simulink model "model_5_exact"  (R2021b)
settings: Solver=VariableStepAuto  StartTime=0.0  StopTime=4e8
values from neighbouring files (symbols this model uses):
  att_Gains = [1 1 1]    [initial_sim2.m]
  Force_Vectors = [Force_Vectors;normal_vector]    [ellip_force_test.m]    (also in initial_sim.m = Force_Vectors'; initial_sim2.m = Force_Vectors'; multi_sim.m = Force_Vectors'; multi_sim2.m = Force_Vectors')
  max_f = 100000    [initial_sim.m]    (also in initial_sim2.m = 10)
  max_M_available = max_M_available*0.7    [initial_sim.m]    (also in initial_sim2.m; multi_sim.m; multi_sim2.m)
  mee_0 = oe2mee([a_0 e_0 incl_0 omega_0 RA_0 theta_0],p.mu)'    [Sample_OT.m]    (also in initial_sim.m = oe2mee(oe_0,params.mu)'; initial_sim2.m = oe2mp(oe_0))
  mee_f = oe2mee([a_f e_f incl_f omega_f RA_f theta_f],p.mu)'    [Sample_OT.m]    (also in initial_sim.m = oe2mee(oe_f,params.mu)'; initial_sim2.m = oe2mp(oe_f))
  Moment_Vectors = [Moment_Vectors;cross([x y z],normal_vector)]    [ellip_force_test.m]    (also in initial_sim.m = Moment_Vectors'; initial_sim2.m = Moment_Vectors'; multi_sim.m = Moment_Vectors'; multi_sim2.m = Moment_Vectors')
  N_sat = length(azimuths)    [ellip_force_test.m]    (also in initial_sim.m = 30; initial_sim2.m = 25; multi_sim.m = sim_data.N_sat; multi_sim2.m = sim_data.N_sat)
  params = 0    [Combo_OT.m]
  R_stop = 1e-2    (= 0.01)    [initial_sim2.m]
  rot_Gains = [1 1 1]    [initial_sim2.m]    (also in multi_sim2.m = inputArg(i_par,4*N_sat+6:4*N_sat+8))
  W = [6.4966    2.6843    0.7051    1.8764    3.9369]    [initial_sim2.m]    (also in lambert_pro.m = 4/(4 - Td); multi_sim2.m = inputArg(i_par,4*N_sat+1:4*N_sat+5))
undefined symbols (not defined in the file or in its folder): t_wait
libraries: slpidlib x6, simulink x3, shared6dof x2
settings Model: Creator=Mehdi  LastModifiedBy=Mehdi
settings DebuggingCC: AlgebraicLoopMsg=none

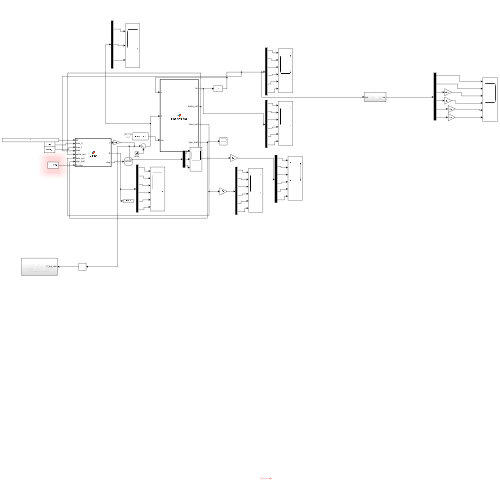
[thumbnail: Simulink's stored preview of the top-level diagram]
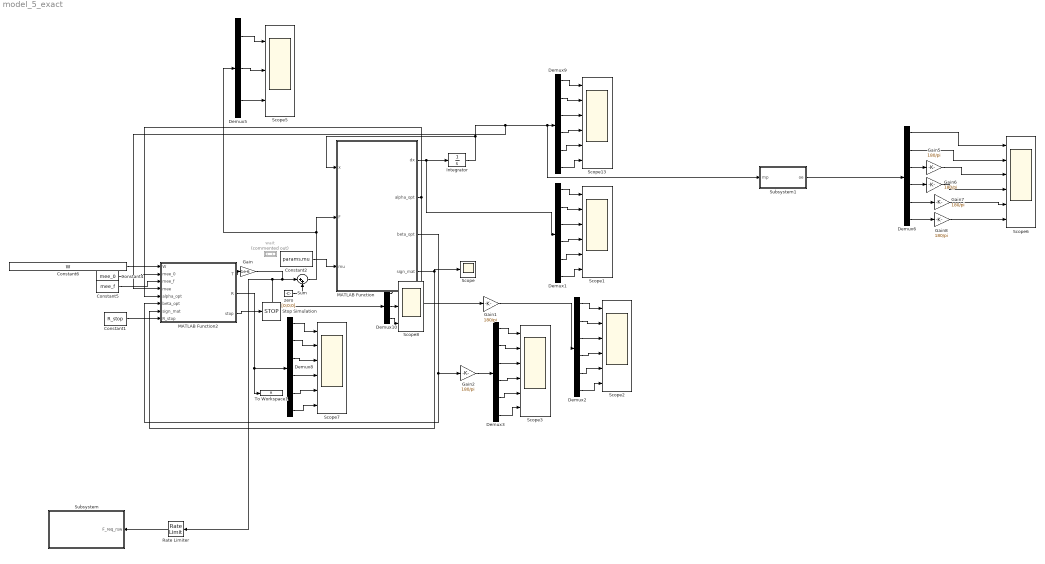
== system model_5_exact ==
  Constant1 : Constant  Value=R_stop
  Constant2 : Constant  Value=params.mu
  Constant4 : Constant  Value=mee_0
  Constant5 : Constant  Value=mee_f
  Constant6 : Constant  Value=W
  Demux{1..3,6,8..9} (6 alike) : Demux  Outputs=6
  Demux10 : Demux  Outputs=3
  Demux5 : Demux  Outputs=3
  Gain : Gain  Gain=1e-6
  Gain{1..2,5..8} (6 alike) : Gain  Gain=180/pi
  Integrator : Integrator  InitialCondition=mee_0
  MATLAB Function : MATLAB Function  TreatAsAtomicUnit=on
  MATLAB Function2 : MATLAB Function  TreatAsAtomicUnit=on
  Rate Limiter : RateLimiter  RisingSlewLimit=1e-5  FallingSlewLimit=-1e-5  SampleTimeMode=inherited
  Scope : Scope
  Scope{1..3,6..7,13} (6 alike) : Scope  NumInputPorts=6
  Scope5 : Scope  NumInputPorts=3
  Scope8 : Scope  NumInputPorts=3
  Stop Simulation : Stop
  Subsystem : Subsystem
  Subsystem1 : Subsystem
  Sum : Sum  Inputs=|++
  To Workspace1 : ToWorkspace  VariableName=R  SaveFormat=Timeseries  SampleTime=-1
      settings: MaxDataPoints=1
  wait : Subsystem  Commented=on
  zero : Constant  Value=[0;0;0]
  wires:
  Integrator/1 -> MATLAB Function2/4(mee), Subsystem1/1(mp), Demux9/1, MATLAB Function/1(x)
  Constant2/1 -> MATLAB Function/3(mu)
  Demux9/5 -> Scope13/5
  Demux9/1 -> Scope13/1
  Demux9/4 -> Scope13/4
  Demux9/3 -> Scope13/3
  Demux9/2 -> Scope13/2
  Demux9/6 -> Scope13/6
  Demux1/6 -> Scope1/6
  Demux1/2 -> Scope1/2
  Demux1/3 -> Scope1/3
  Demux1/4 -> Scope1/4
  Demux1/1 -> Scope1/1
  Demux1/5 -> Scope1/5
  Demux2/6 -> Scope2/6
  Demux2/2 -> Scope2/2
  Demux2/3 -> Scope2/3
  Demux2/4 -> Scope2/4
  Demux2/1 -> Scope2/1
  Demux2/5 -> Scope2/5
  MATLAB Function/2(alpha_opt) -> MATLAB Function2/5(alpha_opt), Gain1/1
  MATLAB Function/3(beta_opt) -> MATLAB Function2/6(beta_opt), Gain2/1
  Demux3/5 -> Scope3/5
  Demux3/1 -> Scope3/1
  Demux3/4 -> Scope3/4
  Demux3/3 -> Scope3/3
  Demux3/2 -> Scope3/2
  Demux3/6 -> Scope3/6
  Constant4/1 -> MATLAB Function2/2(mee_0)
  Constant5/1 -> MATLAB Function2/3(mee_f)
  Constant6/1 -> MATLAB Function2/1(W)
  Demux5/3 -> Scope5/3
  Demux5/2 -> Scope5/2
  Demux5/1 -> Scope5/1
  MATLAB Function2/1(T) -> Gain/1
  zero/1 -> Sum/2
  MATLAB Function2/3(stop) -> Stop Simulation/1
  Demux6/6 -> Gain8/1
  Demux6/3 -> Gain5/1
  Demux6/4 -> Gain6/1
  Demux6/5 -> Gain7/1
  Demux8/4 -> Scope7/4
  Demux8/3 -> Scope7/3
  Demux8/5 -> Scope7/5
  Demux8/2 -> Scope7/2
  Demux8/6 -> Scope7/6
  Demux8/1 -> Scope7/1
  MATLAB Function2/2(R) -> To Workspace1/1, Demux8/1
  Gain1/1 -> Demux2/1
  MATLAB Function/1(dx) -> Demux1/1, Integrator/1
  Gain2/1 -> Demux3/1
  Demux6/1 -> Scope6/1
  Demux6/2 -> Scope6/2
  Gain5/1 -> Scope6/3
  Gain6/1 -> Scope6/4
  Gain7/1 -> Scope6/5
  Gain8/1 -> Scope6/6
  Demux10/2 -> Scope8/2
  Demux10/1 -> Scope8/1
  Demux10/3 -> Scope8/3
  ? -> ?
  Sum/1 -> MATLAB Function/2(F), Demux5/1
  MATLAB Function/4(sign_mat) -> Scope/1, MATLAB Function2/7(sign_mat)
  Rate Limiter/1 -> Subsystem/1(F_req_rsw)
  Subsystem1/1(oe) -> Demux6/1
  Gain/1 -> Rate Limiter/1, Demux10/1, Sum/1
  Constant1/1 -> MATLAB Function2/8(R_stop)

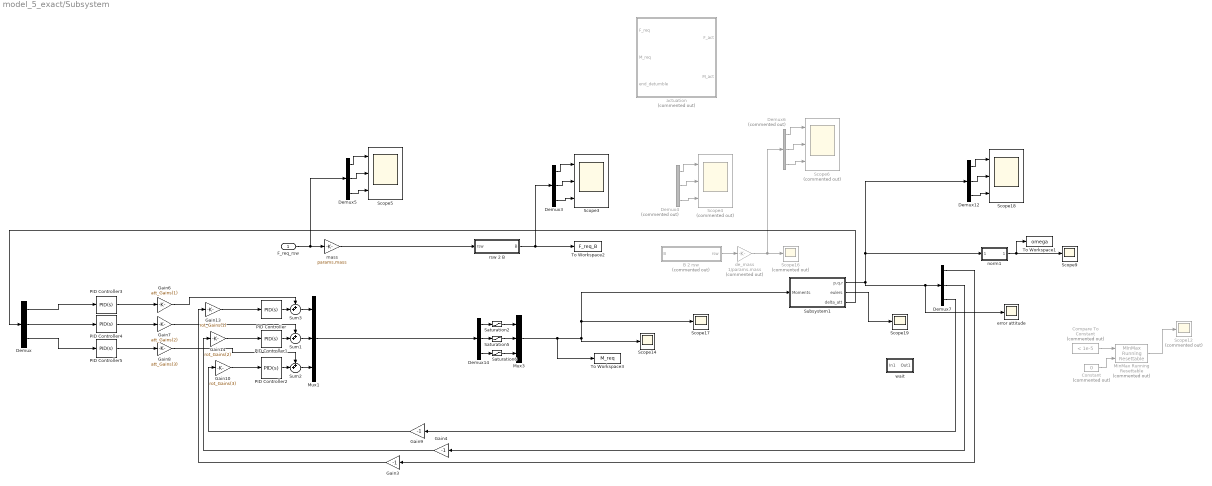
== system model_5_exact/Subsystem ==
  F_req_rsw : Inport
  B 2 rsw : Subsystem  Commented=on
  Compare To Constant : simulink/Logic and Bit Operations/Compare To Constant  Commented=on  relop=<  const=1e-5  OutDataTypeStr=boolean
  Constant : Constant  Commented=on  Value=0
  Demux{,3,5,7,12,14} (6 alike) : Demux  Outputs=3
  Demux4 : Demux  Commented=on  Outputs=3
  Demux6 : Demux  Commented=on  Outputs=3
  Gain10 : Gain  Gain=rot_Gains(3)
  Gain13 : Gain  Gain=rot_Gains(1)
  Gain14 : Gain  Gain=rot_Gains(2)
  Gain3 : Gain  Gain=-1
  Gain4 : Gain  Gain=-1
  Gain6 : Gain  Gain=att_Gains(1)
  Gain7 : Gain  Gain=att_Gains(2)
  Gain8 : Gain  Gain=att_Gains(3)
  Gain9 : Gain  Gain=-1
  MinMax Running Resettable : simulink/Math Operations/MinMax Running Resettable  Commented=on  Function=max  vinit=0.0
  Mux1 : Mux  Inputs=3
  Mux3 : Mux  Inputs=3
  PID Controller : slpidlib/PID Controller  Controller=PID  Form=Parallel  TimeDomain=Continuous-time  UseExternalTs=off  SampleTime=-1  IntegratorMethod=Forward Euler  FilterMethod=Forward Euler  ControllerParametersSource=internal  P=46047.8602202051  I=0.386669360831826  D=-40642086.1977214  UseFilter=on  N=0.0011330092652278  TunerSelectOption=Transfer Function Based (PID Tuner App)  InitialConditionSource=internal  InitialConditionForIntegrator=0  InitialConditionForFilter=0  DifferentiatorICPrevScaledInput=0  ExternalReset=none  TrackingMode=off  Kt=1  LimitOutput=off  SatLimitsSource=internal  UpperSaturationLimit=inf  LowerSaturationLimit=-inf  LinearizeAsGain=on  AntiWindupMode=none  Kb=1  POutMin=[]  POutMax=[]  IOutMin=[]  IOutMax=[]  DOutMin=[]  DOutMax=[]  NOutMin=[]  NOutMax=[]  SumOutMin=[]  SumOutMax=[]  SaturationOutMin=[]  SaturationOutMax=[]  PParamMin=[]  PParamMax=[]  IParamMin=[]  IParamMax=[]  DParamMin=[]  DParamMax=[]  NParamMin=[]  NParamMax=[]  KbParamMin=[]  KbParamMax=[]  KtParamMin=[]  KtParamMax=[]  KbOutMin=[]  KbOutMax=[]  KtOutMin=[]  KtOutMax=[]  IntegratorOutMin=[]  IntegratorOutMax=[]  FilterOutMin=[]  FilterOutMax=[]  SumI1OutMin=[]  SumI1OutMax=[]  SumI2OutMin=[]  SumI2OutMax=[]  SumI3OutMin=[]  SumI3OutMax=[]  SumI4OutMin=[]  SumI4OutMax=[]  SumDOutMin=[]  SumDOutMax=[]  DifferentiatorOutMin=[]  DifferentiatorOutMax=[]  FilterDiffOutCoefMin=[]  FilterDiffOutCoefMax=[]  ReciprocalOutMin=[]  ReciprocalOutMax=[]  SumDenOutMin=[]  SumDenOutMax=[]  SumNumOutMin=[]  SumNumOutMax=[]  DivideOutMin=[]  DivideOutMax=[]  UdiffTsProdOutMin=[]  UdiffTsProdOutMax=[]  NTsProdOutMin=[]  NTsProdOutMax=[]  UintegralTsProdOutMin=[]  UintegralTsProdOutMax=[]  UngainTsProdOutMin=[]  UngainTsProdOutMax=[]  IntegratorContinuousStateAttributes=''  IntegratorStateMustResolveToSignalObject=off  IntegratorRTWStateStorageClass=Auto  FilterContinuousStateAttributes=''  FilterStateMustResolveToSignalObject=off  FilterRTWStateStorageClass=Auto  ParallelPVariant=InternalParameters  IdealPVariant=Disabled  IVariant=InternalParameters  DVariant=InternalParameters  IntegratorVariant=Continuous  SatVariant=Disabled  AWVariant=Passthrough  PCopyVariant=Disabled  TRVariant=Disabled  FdbkBlocksVariant=Forward  IdealPFdbkVariant=Disabled  SatFdbkVariant=Disabled  DerivativeFilterVariant=ContFilter  NVariant=InternalParameters  NCopyVariant=Disabled  FilterICVariant=InternalICsFilter  IntegratorICVariant=InternalICs  ExternalResetVariant=Disabled  TRSumVariant=Passthrough  SumFdbkVariant=Disabled  SumVariant=Sum_PID  TsampFilterVariant=InternalTs  TsampNgainVariant=Passthrough  TsampIntegralVariant=Passthrough  ExternalSaturationOutDataTypeStr=Inherit: Same as second input
  PID Controller1 : slpidlib/PID Controller  Controller=PID  Form=Parallel  TimeDomain=Continuous-time  UseExternalTs=off  SampleTime=-1  IntegratorMethod=Forward Euler  FilterMethod=Forward Euler  ControllerParametersSource=internal  P=22665.0700482182  I=0.192665771971189  D=-23536701.4498255  UseFilter=on  N=0.00096296713864237  TunerSelectOption=Transfer Function Based (PID Tuner App)  InitialConditionSource=internal  InitialConditionForIntegrator=0  InitialConditionForFilter=0  DifferentiatorICPrevScaledInput=0  ExternalReset=none  TrackingMode=off  Kt=1  LimitOutput=off  SatLimitsSource=internal  UpperSaturationLimit=inf  LowerSaturationLimit=-inf  LinearizeAsGain=on  AntiWindupMode=none  Kb=1  POutMin=[]  POutMax=[]  IOutMin=[]  IOutMax=[]  DOutMin=[]  DOutMax=[]  NOutMin=[]  NOutMax=[]  SumOutMin=[]  SumOutMax=[]  SaturationOutMin=[]  SaturationOutMax=[]  PParamMin=[]  PParamMax=[]  IParamMin=[]  IParamMax=[]  DParamMin=[]  DParamMax=[]  NParamMin=[]  NParamMax=[]  KbParamMin=[]  KbParamMax=[]  KtParamMin=[]  KtParamMax=[]  KbOutMin=[]  KbOutMax=[]  KtOutMin=[]  KtOutMax=[]  IntegratorOutMin=[]  IntegratorOutMax=[]  FilterOutMin=[]  FilterOutMax=[]  SumI1OutMin=[]  SumI1OutMax=[]  SumI2OutMin=[]  SumI2OutMax=[]  SumI3OutMin=[]  SumI3OutMax=[]  SumI4OutMin=[]  SumI4OutMax=[]  SumDOutMin=[]  SumDOutMax=[]  DifferentiatorOutMin=[]  DifferentiatorOutMax=[]  FilterDiffOutCoefMin=[]  FilterDiffOutCoefMax=[]  ReciprocalOutMin=[]  ReciprocalOutMax=[]  SumDenOutMin=[]  SumDenOutMax=[]  SumNumOutMin=[]  SumNumOutMax=[]  DivideOutMin=[]  DivideOutMax=[]  UdiffTsProdOutMin=[]  UdiffTsProdOutMax=[]  NTsProdOutMin=[]  NTsProdOutMax=[]  UintegralTsProdOutMin=[]  UintegralTsProdOutMax=[]  UngainTsProdOutMin=[]  UngainTsProdOutMax=[]  IntegratorContinuousStateAttributes=''  IntegratorStateMustResolveToSignalObject=off  IntegratorRTWStateStorageClass=Auto  FilterContinuousStateAttributes=''  FilterStateMustResolveToSignalObject=off  FilterRTWStateStorageClass=Auto  ParallelPVariant=InternalParameters  IdealPVariant=Disabled  IVariant=InternalParameters  DVariant=InternalParameters  IntegratorVariant=Continuous  SatVariant=Disabled  AWVariant=Passthrough  PCopyVariant=Disabled  TRVariant=Disabled  FdbkBlocksVariant=Forward  IdealPFdbkVariant=Disabled  SatFdbkVariant=Disabled  DerivativeFilterVariant=ContFilter  NVariant=InternalParameters  NCopyVariant=Disabled  FilterICVariant=InternalICsFilter  IntegratorICVariant=InternalICs  ExternalResetVariant=Disabled  TRSumVariant=Passthrough  SumFdbkVariant=Disabled  SumVariant=Sum_PID  TsampFilterVariant=InternalTs  TsampNgainVariant=Passthrough  TsampIntegralVariant=Passthrough  ExternalSaturationOutDataTypeStr=Inherit: Same as second input
  PID Controller2 : slpidlib/PID Controller  Controller=PID  Form=Parallel  TimeDomain=Continuous-time  UseExternalTs=off  SampleTime=-1  IntegratorMethod=Forward Euler  FilterMethod=Forward Euler  ControllerParametersSource=internal  P=57156.0298545842  I=0.0195126142821294  D=-17592936910.7499  UseFilter=on  N=3.24050294010588e-06  TunerSelectOption=Transfer Function Based (PID Tuner App)  InitialConditionSource=internal  InitialConditionForIntegrator=0  InitialConditionForFilter=0  DifferentiatorICPrevScaledInput=0  ExternalReset=none  TrackingMode=off  Kt=1  LimitOutput=off  SatLimitsSource=internal  UpperSaturationLimit=inf  LowerSaturationLimit=-inf  LinearizeAsGain=on  AntiWindupMode=none  Kb=1  POutMin=[]  POutMax=[]  IOutMin=[]  IOutMax=[]  DOutMin=[]  DOutMax=[]  NOutMin=[]  NOutMax=[]  SumOutMin=[]  SumOutMax=[]  SaturationOutMin=[]  SaturationOutMax=[]  PParamMin=[]  PParamMax=[]  IParamMin=[]  IParamMax=[]  DParamMin=[]  DParamMax=[]  NParamMin=[]  NParamMax=[]  KbParamMin=[]  KbParamMax=[]  KtParamMin=[]  KtParamMax=[]  KbOutMin=[]  KbOutMax=[]  KtOutMin=[]  KtOutMax=[]  IntegratorOutMin=[]  IntegratorOutMax=[]  FilterOutMin=[]  FilterOutMax=[]  SumI1OutMin=[]  SumI1OutMax=[]  SumI2OutMin=[]  SumI2OutMax=[]  SumI3OutMin=[]  SumI3OutMax=[]  SumI4OutMin=[]  SumI4OutMax=[]  SumDOutMin=[]  SumDOutMax=[]  DifferentiatorOutMin=[]  DifferentiatorOutMax=[]  FilterDiffOutCoefMin=[]  FilterDiffOutCoefMax=[]  ReciprocalOutMin=[]  ReciprocalOutMax=[]  SumDenOutMin=[]  SumDenOutMax=[]  SumNumOutMin=[]  SumNumOutMax=[]  DivideOutMin=[]  DivideOutMax=[]  UdiffTsProdOutMin=[]  UdiffTsProdOutMax=[]  NTsProdOutMin=[]  NTsProdOutMax=[]  UintegralTsProdOutMin=[]  UintegralTsProdOutMax=[]  UngainTsProdOutMin=[]  UngainTsProdOutMax=[]  IntegratorContinuousStateAttributes=''  IntegratorStateMustResolveToSignalObject=off  IntegratorRTWStateStorageClass=Auto  FilterContinuousStateAttributes=''  FilterStateMustResolveToSignalObject=off  FilterRTWStateStorageClass=Auto  ParallelPVariant=InternalParameters  IdealPVariant=Disabled  IVariant=InternalParameters  DVariant=InternalParameters  IntegratorVariant=Continuous  SatVariant=Disabled  AWVariant=Passthrough  PCopyVariant=Disabled  TRVariant=Disabled  FdbkBlocksVariant=Forward  IdealPFdbkVariant=Disabled  SatFdbkVariant=Disabled  DerivativeFilterVariant=ContFilter  NVariant=InternalParameters  NCopyVariant=Disabled  FilterICVariant=InternalICsFilter  IntegratorICVariant=InternalICs  ExternalResetVariant=Disabled  TRSumVariant=Passthrough  SumFdbkVariant=Disabled  SumVariant=Sum_PID  TsampFilterVariant=InternalTs  TsampNgainVariant=Passthrough  TsampIntegralVariant=Passthrough  ExternalSaturationOutDataTypeStr=Inherit: Same as second input
  PID Controller3 : slpidlib/PID Controller  Controller=PID  Form=Parallel  TimeDomain=Continuous-time  UseExternalTs=off  SampleTime=-1  IntegratorMethod=Forward Euler  FilterMethod=Forward Euler  ControllerParametersSource=internal  P=7.2870758510925  I=4.81330185008632e-05  D=272296.627551547  UseFilter=on  N=0.00293249740535471  TunerSelectOption=Transfer Function Based (PID Tuner App)  InitialConditionSource=internal  InitialConditionForIntegrator=0  InitialConditionForFilter=0  DifferentiatorICPrevScaledInput=0  ExternalReset=none  TrackingMode=off  Kt=1  LimitOutput=off  SatLimitsSource=internal  UpperSaturationLimit=inf  LowerSaturationLimit=-inf  LinearizeAsGain=on  AntiWindupMode=none  Kb=1  POutMin=[]  POutMax=[]  IOutMin=[]  IOutMax=[]  DOutMin=[]  DOutMax=[]  NOutMin=[]  NOutMax=[]  SumOutMin=[]  SumOutMax=[]  SaturationOutMin=[]  SaturationOutMax=[]  PParamMin=[]  PParamMax=[]  IParamMin=[]  IParamMax=[]  DParamMin=[]  DParamMax=[]  NParamMin=[]  NParamMax=[]  KbParamMin=[]  KbParamMax=[]  KtParamMin=[]  KtParamMax=[]  KbOutMin=[]  KbOutMax=[]  KtOutMin=[]  KtOutMax=[]  IntegratorOutMin=[]  IntegratorOutMax=[]  FilterOutMin=[]  FilterOutMax=[]  SumI1OutMin=[]  SumI1OutMax=[]  SumI2OutMin=[]  SumI2OutMax=[]  SumI3OutMin=[]  SumI3OutMax=[]  SumI4OutMin=[]  SumI4OutMax=[]  SumDOutMin=[]  SumDOutMax=[]  DifferentiatorOutMin=[]  DifferentiatorOutMax=[]  FilterDiffOutCoefMin=[]  FilterDiffOutCoefMax=[]  ReciprocalOutMin=[]  ReciprocalOutMax=[]  SumDenOutMin=[]  SumDenOutMax=[]  SumNumOutMin=[]  SumNumOutMax=[]  DivideOutMin=[]  DivideOutMax=[]  UdiffTsProdOutMin=[]  UdiffTsProdOutMax=[]  NTsProdOutMin=[]  NTsProdOutMax=[]  UintegralTsProdOutMin=[]  UintegralTsProdOutMax=[]  UngainTsProdOutMin=[]  UngainTsProdOutMax=[]  IntegratorContinuousStateAttributes=''  IntegratorStateMustResolveToSignalObject=off  IntegratorRTWStateStorageClass=Auto  FilterContinuousStateAttributes=''  FilterStateMustResolveToSignalObject=off  FilterRTWStateStorageClass=Auto  ParallelPVariant=InternalParameters  IdealPVariant=Disabled  IVariant=InternalParameters  DVariant=InternalParameters  IntegratorVariant=Continuous  SatVariant=Disabled  AWVariant=Passthrough  PCopyVariant=Disabled  TRVariant=Disabled  FdbkBlocksVariant=Forward  IdealPFdbkVariant=Disabled  SatFdbkVariant=Disabled  DerivativeFilterVariant=ContFilter  NVariant=InternalParameters  NCopyVariant=Disabled  FilterICVariant=InternalICsFilter  IntegratorICVariant=InternalICs  ExternalResetVariant=Disabled  TRSumVariant=Passthrough  SumFdbkVariant=Disabled  SumVariant=Sum_PID  TsampFilterVariant=InternalTs  TsampNgainVariant=Passthrough  TsampIntegralVariant=Passthrough  ExternalSaturationOutDataTypeStr=Inherit: Same as second input
  PID Controller4 : slpidlib/PID Controller  Controller=PID  Form=Parallel  TimeDomain=Continuous-time  UseExternalTs=off  SampleTime=-1  IntegratorMethod=Forward Euler  FilterMethod=Forward Euler  ControllerParametersSource=internal  P=7.2870758510925  I=4.81330185008632e-05  D=272296.627551547  UseFilter=on  N=0.00293249740535471  TunerSelectOption=Transfer Function Based (PID Tuner App)  InitialConditionSource=internal  InitialConditionForIntegrator=0  InitialConditionForFilter=0  DifferentiatorICPrevScaledInput=0  ExternalReset=none  TrackingMode=off  Kt=1  LimitOutput=off  SatLimitsSource=internal  UpperSaturationLimit=inf  LowerSaturationLimit=-inf  LinearizeAsGain=on  AntiWindupMode=none  Kb=1  POutMin=[]  POutMax=[]  IOutMin=[]  IOutMax=[]  DOutMin=[]  DOutMax=[]  NOutMin=[]  NOutMax=[]  SumOutMin=[]  SumOutMax=[]  SaturationOutMin=[]  SaturationOutMax=[]  PParamMin=[]  PParamMax=[]  IParamMin=[]  IParamMax=[]  DParamMin=[]  DParamMax=[]  NParamMin=[]  NParamMax=[]  KbParamMin=[]  KbParamMax=[]  KtParamMin=[]  KtParamMax=[]  KbOutMin=[]  KbOutMax=[]  KtOutMin=[]  KtOutMax=[]  IntegratorOutMin=[]  IntegratorOutMax=[]  FilterOutMin=[]  FilterOutMax=[]  SumI1OutMin=[]  SumI1OutMax=[]  SumI2OutMin=[]  SumI2OutMax=[]  SumI3OutMin=[]  SumI3OutMax=[]  SumI4OutMin=[]  SumI4OutMax=[]  SumDOutMin=[]  SumDOutMax=[]  DifferentiatorOutMin=[]  DifferentiatorOutMax=[]  FilterDiffOutCoefMin=[]  FilterDiffOutCoefMax=[]  ReciprocalOutMin=[]  ReciprocalOutMax=[]  SumDenOutMin=[]  SumDenOutMax=[]  SumNumOutMin=[]  SumNumOutMax=[]  DivideOutMin=[]  DivideOutMax=[]  UdiffTsProdOutMin=[]  UdiffTsProdOutMax=[]  NTsProdOutMin=[]  NTsProdOutMax=[]  UintegralTsProdOutMin=[]  UintegralTsProdOutMax=[]  UngainTsProdOutMin=[]  UngainTsProdOutMax=[]  IntegratorContinuousStateAttributes=''  IntegratorStateMustResolveToSignalObject=off  IntegratorRTWStateStorageClass=Auto  FilterContinuousStateAttributes=''  FilterStateMustResolveToSignalObject=off  FilterRTWStateStorageClass=Auto  ParallelPVariant=InternalParameters  IdealPVariant=Disabled  IVariant=InternalParameters  DVariant=InternalParameters  IntegratorVariant=Continuous  SatVariant=Disabled  AWVariant=Passthrough  PCopyVariant=Disabled  TRVariant=Disabled  FdbkBlocksVariant=Forward  IdealPFdbkVariant=Disabled  SatFdbkVariant=Disabled  DerivativeFilterVariant=ContFilter  NVariant=InternalParameters  NCopyVariant=Disabled  FilterICVariant=InternalICsFilter  IntegratorICVariant=InternalICs  ExternalResetVariant=Disabled  TRSumVariant=Passthrough  SumFdbkVariant=Disabled  SumVariant=Sum_PID  TsampFilterVariant=InternalTs  TsampNgainVariant=Passthrough  TsampIntegralVariant=Passthrough  ExternalSaturationOutDataTypeStr=Inherit: Same as second input
  PID Controller5 : slpidlib/PID Controller  Controller=PID  Form=Parallel  TimeDomain=Continuous-time  UseExternalTs=off  SampleTime=-1  IntegratorMethod=Forward Euler  FilterMethod=Forward Euler  ControllerParametersSource=internal  P=7.2870758510925  I=4.81330185008632e-05  D=272296.627551547  UseFilter=on  N=0.00293249740535471  TunerSelectOption=Transfer Function Based (PID Tuner App)  InitialConditionSource=internal  InitialConditionForIntegrator=0  InitialConditionForFilter=0  DifferentiatorICPrevScaledInput=0  ExternalReset=none  TrackingMode=off  Kt=1  LimitOutput=off  SatLimitsSource=internal  UpperSaturationLimit=inf  LowerSaturationLimit=-inf  LinearizeAsGain=on  AntiWindupMode=none  Kb=1  POutMin=[]  POutMax=[]  IOutMin=[]  IOutMax=[]  DOutMin=[]  DOutMax=[]  NOutMin=[]  NOutMax=[]  SumOutMin=[]  SumOutMax=[]  SaturationOutMin=[]  SaturationOutMax=[]  PParamMin=[]  PParamMax=[]  IParamMin=[]  IParamMax=[]  DParamMin=[]  DParamMax=[]  NParamMin=[]  NParamMax=[]  KbParamMin=[]  KbParamMax=[]  KtParamMin=[]  KtParamMax=[]  KbOutMin=[]  KbOutMax=[]  KtOutMin=[]  KtOutMax=[]  IntegratorOutMin=[]  IntegratorOutMax=[]  FilterOutMin=[]  FilterOutMax=[]  SumI1OutMin=[]  SumI1OutMax=[]  SumI2OutMin=[]  SumI2OutMax=[]  SumI3OutMin=[]  SumI3OutMax=[]  SumI4OutMin=[]  SumI4OutMax=[]  SumDOutMin=[]  SumDOutMax=[]  DifferentiatorOutMin=[]  DifferentiatorOutMax=[]  FilterDiffOutCoefMin=[]  FilterDiffOutCoefMax=[]  ReciprocalOutMin=[]  ReciprocalOutMax=[]  SumDenOutMin=[]  SumDenOutMax=[]  SumNumOutMin=[]  SumNumOutMax=[]  DivideOutMin=[]  DivideOutMax=[]  UdiffTsProdOutMin=[]  UdiffTsProdOutMax=[]  NTsProdOutMin=[]  NTsProdOutMax=[]  UintegralTsProdOutMin=[]  UintegralTsProdOutMax=[]  UngainTsProdOutMin=[]  UngainTsProdOutMax=[]  IntegratorContinuousStateAttributes=''  IntegratorStateMustResolveToSignalObject=off  IntegratorRTWStateStorageClass=Auto  FilterContinuousStateAttributes=''  FilterStateMustResolveToSignalObject=off  FilterRTWStateStorageClass=Auto  ParallelPVariant=InternalParameters  IdealPVariant=Disabled  IVariant=InternalParameters  DVariant=InternalParameters  IntegratorVariant=Continuous  SatVariant=Disabled  AWVariant=Passthrough  PCopyVariant=Disabled  TRVariant=Disabled  FdbkBlocksVariant=Forward  IdealPFdbkVariant=Disabled  SatFdbkVariant=Disabled  DerivativeFilterVariant=ContFilter  NVariant=InternalParameters  NCopyVariant=Disabled  FilterICVariant=InternalICsFilter  IntegratorICVariant=InternalICs  ExternalResetVariant=Disabled  TRSumVariant=Passthrough  SumFdbkVariant=Disabled  SumVariant=Sum_PID  TsampFilterVariant=InternalTs  TsampNgainVariant=Passthrough  TsampIntegralVariant=Passthrough  ExternalSaturationOutDataTypeStr=Inherit: Same as second input
  Saturation2 : Saturate  UpperLimit=max_M_available(1,1)  LowerLimit=max_M_available(1,2)
  Saturation5 : Saturate  UpperLimit=max_M_available(2,1)  LowerLimit=max_M_available(2,2)
  Saturation6 : Saturate  UpperLimit=max_M_available(3,1)  LowerLimit=max_M_available(3,2)
  Scope12 : Scope  Commented=on
  Scope{9,14,17,19} (4 alike) : Scope
  Scope16 : Scope  Commented=on
  Scope18 : Scope  NumInputPorts=3
  Scope3 : Scope  NumInputPorts=3
  Scope4 : Scope  Commented=on  NumInputPorts=3
  Scope5 : Scope  NumInputPorts=3
  Scope6 : Scope  Commented=on  NumInputPorts=3
  Subsystem1 : Subsystem
  Sum1 : Sum  Inputs=++|
  Sum2 : Sum  Inputs=++|
  Sum3 : Sum  Inputs=++|
  To Workspace1 : ToWorkspace  VariableName=omega  SaveFormat=Timeseries  SampleTime=-1
      settings: MaxDataPoints=1
  To Workspace2 : ToWorkspace  VariableName=F_req_B  SaveFormat=Timeseries  SampleTime=-1
  To Workspace3 : ToWorkspace  VariableName=M_req  SaveFormat=Timeseries  SampleTime=-1
  actuation : Subsystem  Commented=on
  de_mass : Gain  Commented=on  Gain=1/params.mass
  error attitude : Scope
  mass : Gain  Gain=params.mass
  norm1 : Subsystem
  rsw 2 B : Subsystem
  wait : Subsystem
  wires:
  norm1/1(Out1) -> To Workspace1/1, Scope9/1
  Gain9/1 -> Gain10/1
  Gain3/1 -> Gain13/1
  Mux3/1 -> Subsystem1/1(Moments), Scope17/1, Scope14/1, To Workspace3/1
  B 2 rsw/1(rsw) -> de_mass/1
  Demux7/2 -> Gain4/1
  Saturation5/1 -> Mux3/2
  Gain4/1 -> Gain14/1
  Demux7/3 -> Gain9/1
  Demux14/3 -> Saturation6/1
  Demux12/2 -> Scope18/2
  Saturation2/1 -> Mux3/1
  Demux12/1 -> Scope18/1
  rsw 2 B/1(B) -> To Workspace2/1, Demux3/1
  Subsystem1/2(eulers) -> Scope19/1
  Demux14/1 -> Saturation2/1
  Demux12/3 -> Scope18/3
  Demux14/2 -> Saturation5/1
  MinMax Running Resettable/1 -> Scope12/1
  Compare To Constant/1 -> MinMax Running Resettable/1
  Constant/1 -> MinMax Running Resettable/2
  Demux7/1 -> Gain3/1
  Saturation6/1 -> Mux3/3
  Demux3/3 -> Scope3/3
  Demux3/1 -> Scope3/1
  Demux3/2 -> Scope3/2
  Demux4/2 -> Scope4/2
  Demux4/1 -> Scope4/1
  Demux4/3 -> Scope4/3
  F_req_rsw/1 -> Demux5/1, mass/1
  Demux5/2 -> Scope5/2
  Demux5/1 -> Scope5/1
  Demux5/3 -> Scope5/3
  Demux6/3 -> Scope6/3
  Demux6/1 -> Scope6/1
  Demux6/2 -> Scope6/2
  de_mass/1 -> Demux6/1, Scope16/1
  mass/1 -> rsw 2 B/1(rsw)
  Mux1/1 -> Demux14/1
  Subsystem1/1(p,q,r) -> error attitude/1, Demux7/1, Demux12/1, norm1/1(p,q,r)
  Subsystem1/3(delta_att) -> Demux/1
  Demux/1 -> PID Controller3/1
  Demux/2 -> PID Controller4/1
  Demux/3 -> PID Controller5/1
  PID Controller3/1 -> Gain6/1
  Gain6/1 -> Sum3/1
  PID Controller4/1 -> Gain7/1
  PID Controller5/1 -> Gain8/1
  PID Controller/1 -> Sum3/2
  Sum3/1 -> Mux1/1
  Gain13/1 -> PID Controller/1
  Gain14/1 -> PID Controller1/1
  Gain10/1 -> PID Controller2/1
  Gain7/1 -> Sum1/1
  Gain8/1 -> Sum2/1
  PID Controller2/1 -> Sum2/2
  Sum2/1 -> Mux1/3
  PID Controller1/1 -> Sum1/2
  Sum1/1 -> Mux1/2

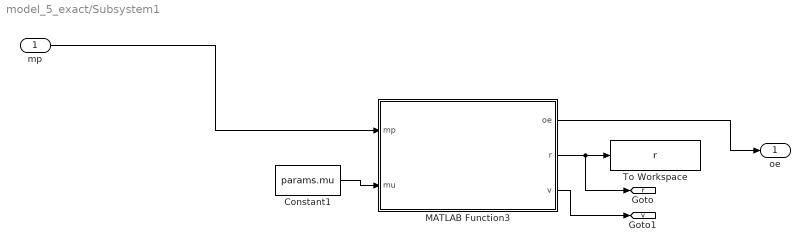
== system model_5_exact/Subsystem1 ==
  mp : Inport
  Constant1 : Constant  Value=params.mu
  MATLAB Function3 : MATLAB Function  TreatAsAtomicUnit=on
  To Workspace : ToWorkspace  VariableName=r  SaveFormat=Timeseries  SampleTime=-1
  oe : Outport
  tag scope: r=global, v=global
  wires:
  Constant1/1 -> MATLAB Function3/2(mu)
  MATLAB Function3/1(oe) -> oe/1
  MATLAB Function3/2(r) -> [r], To Workspace/1
  mp/1 -> MATLAB Function3/1(mp)
  MATLAB Function3/3(v) -> [v]

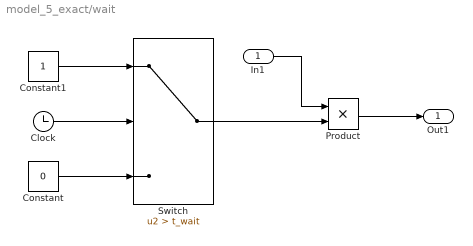
== system model_5_exact/wait ==
  In1 : Inport
  Clock : Clock
  Constant : Constant  Value=0
  Constant1 : Constant
  Product : Product
  Switch : Switch  Criteria=u2 > Threshold  Threshold=t_wait
  Out1 : Outport
  wires:
  Clock/1 -> Switch/2
  Constant1/1 -> Switch/1
  Switch/1 -> Product/2
  Product/1 -> Out1/1
  In1/1 -> Product/1
  Constant/1 -> Switch/3

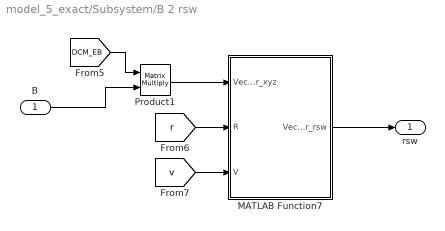
== system model_5_exact/Subsystem/B 2 rsw ==
  B : Inport
  MATLAB Function7 : MATLAB Function  TreatAsAtomicUnit=on
  Product1 : Product  Multiplication=Matrix(*)
  rsw : Outport
  wires:
  Product1/1 -> MATLAB Function7/1(Vector_xyz)
  [v] -> MATLAB Function7/3(V)
  [DCM_EB] -> Product1/1
  [r] -> MATLAB Function7/2(R)
  B/1 -> Product1/2
  MATLAB Function7/1(Vector_rsw) -> rsw/1

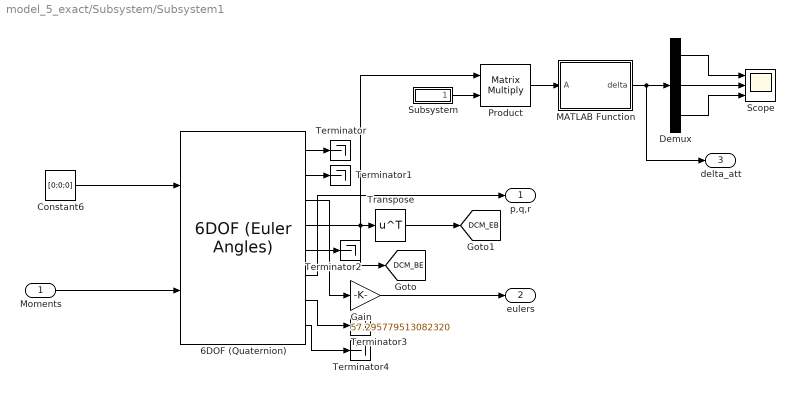
== system model_5_exact/Subsystem/Subsystem1 ==
  Moments : Inport
  6DOF (Quaternion) : shared6dof/6DOF (Euler Angles)  units=Metric (MKS)  mtype=Fixed  rep=Quaternion  xme_0=[0 0 0]  Vm_0=[0 0 0]  eul_0=eul_0  pm_0=pqr_0  mass_0=1.0  mass_e=0.5  mass_f=2.0  inertia=params.Inertia  inertia_e=eye(3)  inertia_f=2*eye(3)  k_quat=1.0  vre_flag=on  abi_flag=off  aMode=0  xme_statename=''  Vm_statename=''  eul_statename=''  quat_statename=''  pm_statename=''  mass_statename=''
      settings: SourceProductBaseCode=AE,PW,DR,MT,UV,VE
  Constant6 : Constant  Value=[0;0;0]
  Demux : Demux  Outputs=3
  Gain : Gain  Gain=57.295779513082320
  MATLAB Function : MATLAB Function  TreatAsAtomicUnit=on
  Product : Product  Multiplication=Matrix(*)
  Scope : Scope  NumInputPorts=3
  Subsystem : Subsystem
  Terminator{,1..4} (5 alike) : Terminator
  Transpose : Math  Operator=transpose  SaturateOnIntegerOverflow=on
  p,q,r : Outport
  eulers : Outport  Port=2
  delta_att : Outport  Port=3
  tag scope: DCM_BE=global, DCM_EB=global
  wires:
  6DOF (Quaternion)/7 -> Terminator3/1
  Constant6/1 -> 6DOF (Quaternion)/1
  6DOF (Quaternion)/3 -> Gain/1
  6DOF (Quaternion)/1 -> Terminator/1
  6DOF (Quaternion)/6 -> p,q,r/1
  6DOF (Quaternion)/5 -> Terminator2/1
  6DOF (Quaternion)/2 -> Terminator1/1
  Gain/1 -> eulers/1
  6DOF (Quaternion)/4 -> Product/1, [DCM_BE], Transpose/1
  6DOF (Quaternion)/8 -> Terminator4/1
  Moments/1 -> 6DOF (Quaternion)/2
  Transpose/1 -> [DCM_EB]
  Product/1 -> MATLAB Function/1(A)
  MATLAB Function/1(delta) -> delta_att/1, Demux/1
  Demux/1 -> Scope/1
  Demux/2 -> Scope/2
  Demux/3 -> Scope/3
  Subsystem/1(DCM_T') -> Product/2

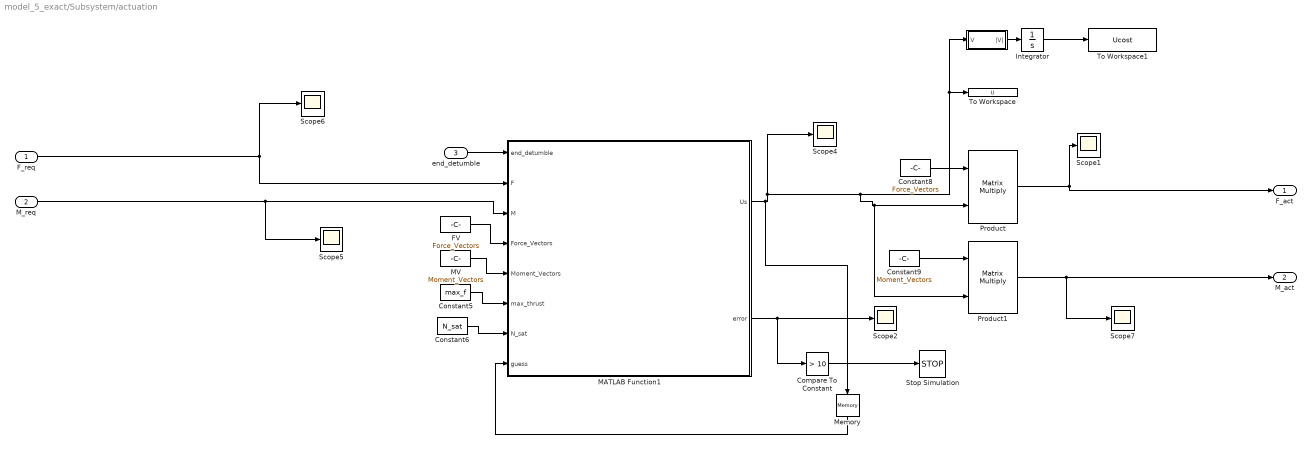
== system model_5_exact/Subsystem/actuation ==
  F_req : Inport
  M_req : Inport  Port=2
  end_detumble : Inport  Port=3
  " " : Subsystem
  Compare To Constant : simulink/Logic and Bit Operations/Compare To Constant  relop=>  const=10  OutDataTypeStr=boolean
  Constant5 : Constant  Value=max_f
  Constant6 : Constant  Value=N_sat
  Constant8 : Constant  Value=Force_Vectors
  Constant9 : Constant  Value=Moment_Vectors
  FV : Constant  Value=Force_Vectors
  Integrator : Integrator
  MATLAB Function1 : MATLAB Function  TreatAsAtomicUnit=on
  MV : Constant  Value=Moment_Vectors
  Memory : Memory  InitialCondition=zeros(N_sat,1)
  Product : Product  Multiplication=Matrix(*)
  Product1 : Product  Multiplication=Matrix(*)
  Scope{1..2,4..7} (6 alike) : Scope
  Stop Simulation : Stop
  To Workspace : ToWorkspace  VariableName=U  SaveFormat=Timeseries  SampleTime=-1
  To Workspace1 : ToWorkspace  VariableName=Ucost  SaveFormat=Timeseries  SampleTime=-1
      settings: MaxDataPoints=1
  F_act : Outport
  M_act : Outport  Port=2
  wires:
  Constant6/1 -> MATLAB Function1/7(N_sat)
  Constant9/1 -> Product1/1
  Memory/1 -> MATLAB Function1/8(guess)
  MATLAB Function1/2(error) -> Compare To Constant/1, Scope2/1
  FV/1 -> MATLAB Function1/4(Force_Vectors)
  MV/1 -> MATLAB Function1/5(Moment_Vectors)
  Product1/1 -> Scope7/1, M_act/1
  Constant8/1 -> Product/1
  Constant5/1 -> MATLAB Function1/6(max_thrust)
  F_req/1 -> MATLAB Function1/2(F), Scope6/1
  Product/1 -> F_act/1, Scope1/1
  end_detumble/1 -> MATLAB Function1/1(end_detumble)
  MATLAB Function1/1(Us) -> Scope4/1, Product/2, Product1/2, " "/1(V), To Workspace/1, Memory/1
  " "/1(|V|) -> Integrator/1
  Integrator/1 -> To Workspace1/1
  M_req/1 -> MATLAB Function1/3(M), Scope5/1
  Compare To Constant/1 -> Stop Simulation/1

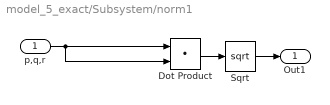
== system model_5_exact/Subsystem/norm1 ==
  p,q,r : Inport
  Dot Product : DotProduct  InputSameDT=on  OutDataTypeStr=Inherit: Inherit via internal rule
  Sqrt : Sqrt  OutputSignalType=real  SaturateOnIntegerOverflow=on
  Out1 : Outport
  wires:
  Dot Product/1 -> Sqrt/1
  p,q,r/1 -> Dot Product/1, Dot Product/2
  Sqrt/1 -> Out1/1

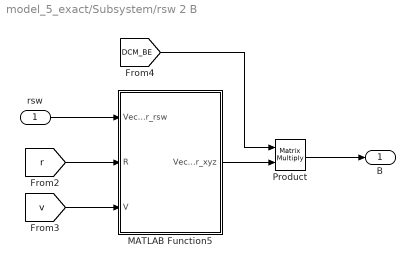
== system model_5_exact/Subsystem/rsw 2 B ==
  rsw : Inport
  MATLAB Function5 : MATLAB Function  TreatAsAtomicUnit=on
  Product : Product  Multiplication=Matrix(*)
  B : Outport
  wires:
  [DCM_BE] -> Product/1
  rsw/1 -> MATLAB Function5/1(Vector_rsw)
  MATLAB Function5/1(Vector_xyz) -> Product/2
  [v] -> MATLAB Function5/3(V)
  [r] -> MATLAB Function5/2(R)
  Product/1 -> B/1

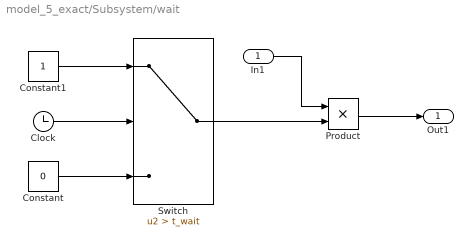
== system model_5_exact/Subsystem/wait ==
  In1 : Inport
  Clock : Clock
  Constant : Constant  Value=0
  Constant1 : Constant
  Product : Product
  Switch : Switch  Criteria=u2 > Threshold  Threshold=t_wait
  Out1 : Outport
  wires:
  Clock/1 -> Switch/2
  Constant1/1 -> Switch/1
  Switch/1 -> Product/2
  Product/1 -> Out1/1
  In1/1 -> Product/1
  Constant/1 -> Switch/3

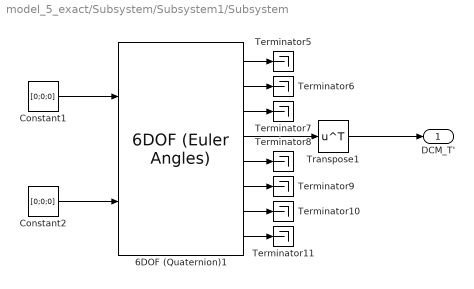
== system model_5_exact/Subsystem/Subsystem1/Subsystem ==
  6DOF (Quaternion)1 : shared6dof/6DOF (Euler Angles)  units=Metric (MKS)  mtype=Fixed  rep=Quaternion  xme_0=[0 0 0]  Vm_0=[0 0 0]  eul_0=target_angles  pm_0=[0 0 0]  mass_0=1.0  mass_e=0.5  mass_f=2.0  inertia=params.Inertia  inertia_e=eye(3)  inertia_f=2*eye(3)  k_quat=1.0  vre_flag=on  abi_flag=off  aMode=0  xme_statename=''  Vm_statename=''  eul_statename=''  quat_statename=''  pm_statename=''  mass_statename=''
      settings: SourceProductBaseCode=AE,PW,DR,MT,UV,VE
  Constant1 : Constant  Value=[0;0;0]
  Constant2 : Constant  Value=[0;0;0]
  Terminator{5..11} (7 alike) : Terminator
  Transpose1 : Math  Operator=transpose  SaturateOnIntegerOverflow=on
  DCM_T' : Outport
  wires:
  6DOF (Quaternion)1/8 -> Terminator11/1
  6DOF (Quaternion)1/3 -> Terminator7/1
  Constant1/1 -> 6DOF (Quaternion)1/1
  6DOF (Quaternion)1/6 -> Terminator9/1
  6DOF (Quaternion)1/1 -> Terminator5/1
  6DOF (Quaternion)1/7 -> Terminator10/1
  Constant2/1 -> 6DOF (Quaternion)1/2
  6DOF (Quaternion)1/5 -> Terminator8/1
  6DOF (Quaternion)1/2 -> Terminator6/1
  6DOF (Quaternion)1/4 -> Transpose1/1
  Transpose1/1 -> DCM_T'/1

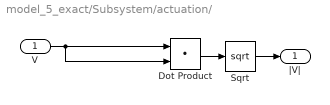
== system model_5_exact/Subsystem/actuation/  ==
  V : Inport
  Dot Product : DotProduct  InputSameDT=on  OutDataTypeStr=Inherit: Inherit via internal rule
  Sqrt : Sqrt  OutputSignalType=real  SaturateOnIntegerOverflow=on
  |V| : Outport
  wires:
  Dot Product/1 -> Sqrt/1
  V/1 -> Dot Product/1, Dot Product/2
  Sqrt/1 -> |V|/1

== matlab function model_5_exact/Subsystem/B 2 rsw/MATLAB Function7 ==
  data: Vector_xyz input; R input; Vector_rsw output; V input
function Vector_rsw=xyz2rsw(Vector_xyz,R,V)

Vector_rsw=zeros(3,1);

e_r=R/norm(R);
h=cross(R,V);
e_w=h/norm(h);
e_s=cross(e_w,e_r);


Vector_rsw(1)=dot(Vector_xyz,e_r);
Vector_rsw(2)=dot(Vector_xyz,e_s);
Vector_rsw(3)=dot(Vector_xyz,e_w);

end

== matlab function model_5_exact/Subsystem/actuation/MATLAB Function1 ==
  data: end_detumble input; F input size=3; Us output; M input size=3; Force_Vectors input; Moment_Vectors input; error output; max_thrust input; N_sat input size=1; guess input
function [Us,error] = cotrol_allocation(end_detumble,F,M,Force_Vectors,Moment_Vectors,max_thrust,N_sat,guess)


maxIter=5;

% Us=zeros(N_sat,1);
% Uss=zeros(N_sat,1);
if end_detumble==0
    %     b=[F(1);F(2);F(3);0;0;0];
    b=[F(1);F(2);F(3);M(1);M(2);M(3)];
else
    b=[F(1);F(2);F(3);0;0;0];
    %     b=[0;0;0;M(1);M(2);M(3)];
end
C=[Force_Vectors;Moment_Vectors];

options = optimoptions('lsqnonlin','Algorithm','levenberg-marquardt','MaxIterations',maxIter);
LB=zeros(N_sat,1);
UB=max_thrust*ones(N_sat,1);
% x0=zeros(N_sat,1);
x0=guess;

% C*x0-b

fun=@(x)(C*x-b);



[Uss,error]=lsqnonlin(fun,x0,LB,UB,options);


if error<1e-4
    
    
    Us=Uss(1:30,1);
    
else
    
    Us=zeros(30,1);
    
end

%
% F_out=Force_Vectors*Us;
% M_out=Moment_Vectors*Us;



% Us=C*x0-b;


% for i=1:N_sat
%     Us(i)=U1(i);
% end

% error=0;


end

== matlab function model_5_exact/MATLAB Function ==
  data: x input; F input; dx output; mu input; alpha_opt output; beta_opt output; sign_mat output
function [dx,alpha_opt,beta_opt,sign_mat] = path_dynamics(x,F,mu)


%%%% to be optimized

% a
% ep1=e*sin(omega+OMEGA);
% ep2=e*cos(omega+OMEGA);
% zig1=tan(inc/2)*sin(OMEGA);
% zig2=tan(inc/2)*cos(OMEGA);
% lambda=theta+omega+OMEGA;


a=x(1);
ep1=x(2);
ep2=x(3);
zig1=x(4);
zig2=x(5);
lambda=x(6);

slam=sin(lambda);
clam=cos(lambda);
L=a*(1-ep1^2-ep2^2);
h=sqrt(mu*L);
r=L/(1+ep1*slam+ep2*clam);

%%% to be optimized!



a_dot_=2*a^2/h*[ep2*slam-ep1*clam L/r 0];
ep1_dot_=r/h*[-L/r*clam ep1+(1+L/r)*slam -ep2*(zig1*clam-zig2*slam)];
ep2_dot_=r/h*[L/r*slam ep2+(1+L/r)*clam ep1*(zig1*clam-zig2*slam)];
zig1_dot_=r/(2*h)*[0 0 (1+zig1^2+zig2^2)*slam];
zig2_dot_=r/(2*h)*[0 0 (1+zig1^2+zig2^2)*clam];
lambda_dot_=r/h*[0 0 zig2*slam-zig1*clam];


a_dot=dot(a_dot_,F);
ep1_dot=dot(ep1_dot_,F);
ep2_dot=dot(ep2_dot_,F);
zig1_dot=dot(zig1_dot_,F);
zig2_dot=dot(zig2_dot_,F);
lambda_dot=h/r^2+dot(lambda_dot_,F);

% % % a_dot=2*a^2/h*dot([ep2*slam-ep1*clam L/r 0],F);
% % % ep1_dot=r/h*dot([-L/r*clam ep1+(1+L/r)*slam -ep2*(zig1*clam-zig2*slam)],F);
% % % ep2_dot=r/h*dot([L/r*slam ep2+(1+L/r)*clam ep1*(zig1*clam-zig2*slam)],F);
% % % zig1_dot=r/(2*h)*dot([0 0 (1+zig1^2+zig2^2)*slam],F);
% % % zig2_dot=r/(2*h)*dot([0 0 (1+zig1^2+zig2^2)*clam],F);
% % % lambda_dot=h/r^2+r/h*dot([0 0 zig2*slam-zig1*clam],F);

% dx=zeros(6,1);

dx=[a_dot;ep1_dot;ep2_dot;zig1_dot;zig2_dot;lambda_dot];


% sign_mat=sign([ep2*slam-ep1*clam L/r 0;-L/r*clam ep1+(1+L/r)*slam -ep2*(zig1*clam-zig2*slam);L/r*slam ep2+(1+L/r)*clam ep1*(zig1*clam-zig2*slam);0 0 (1+zig1^2+zig2^2)*slam;0 0 (1+zig1^2+zig2^2)*clam;0 0 zig2*slam-zig1*clam]);
% sign_mat=sign([ep2*slam-ep1*clam 1 0;-clam ep1+(1+L/r)*slam -ep2*(zig1*clam-zig2*slam);slam ep2+(1+L/r)*clam ep1*(zig1*clam-zig2*slam);0 0 slam;0 0 clam;0 0 zig2*slam-zig1*clam]);



% [a e i omega OMEGA theta]

alpha_opt=zeros(6,1);
beta_opt=zeros(6,1);


%%% based on oe
% % % ep1plus=ep1*slam+ep2*clam;
% % % ep2minus=ep2*slam-ep2*clam;
% % % zig1c=zig1*clam-zig2*slam;
% % % zig2s=zig2*slam-zig1*clam;
% % % alpha_opt(1)=atan((r/L)*ep2minus);
% % % alpha_opt(2)=atan((L/r*ep2minus)/(ep1^2+ep2^2+(1+L/r)*ep1plus));
% % % beta_opt(3)=sign(zig1*slam+zig2*clam)*pi/2;
% % % beta_opt(4)=sign(zig2s)*pi/2;
% % % alpha_opt(5)=atan(-L/(L+r)*(ep1plus/ep2minus));
% % % sinaw=sin(alpha_opt(5));
% % % cosaw=cos(alpha_opt(5));
% % % beta_opt(5)=atan((-(ep1^2+ep2^2)/(zig1^2+zig2^2))*((r*(zig1^2+zig2^2)*zig2s+r/2*(1+zig1^2+zig2^2)*zig1c)/(L*ep1plus*sinaw-(L+r)*ep2minus*cosaw)));
% alpha_opt(6)=atan(-L/(L+r)*ep1plus/ep2minus);
% beta_opt(6)=


alpha_opt(1)=atan(r/L*(ep2*slam-ep1*clam));
alpha_opt(2)=atan(-L*clam/(r*ep1+(r+L)*slam));
alpha_opt(3)=atan(L*slam/(r*ep2+(r+L)*clam));


beta_opt(2)=atan(r*ep2*(zig1*clam-zig2*slam)/(L*clam*sin(alpha_opt(2))-(r*ep1+(r+L)*slam)*cos(alpha_opt(2))));
beta_opt(3)=atan(r*ep1*(zig1*clam-zig2*slam)/(L*slam*sin(alpha_opt(3))-(r*ep2+(r+L)*clam)*cos(alpha_opt(3))));

beta_opt(4)=sign(slam)*pi/2;
beta_opt(5)=sign(clam)*pi/2;

beta_opt(6)=sign(zig2*slam-zig1*clam)*pi/2;


% e=sqrt(ep1^2+ep2^2);
% inc=2*atan(sqrt(zig1^2+zig2^2));
% OMEGA=atan(zig1/zig2);
% omega=atan(ep1/ep2)-OMEGA;
% theta=lambda-atan(ep1/ep2);

% 
% F_sample=zeros(3,6);
% sign_vec=zeros(6,2);

% for i=1:6
%     F_sample(:,i)=[sin(alpha_opt(i))*cos(beta_opt(i));cos(alpha_opt(i))*cos(beta_opt(i));sin(beta_opt(i))];
% end

% for i=1:6
%     F_sample(:,i)=[sin(alpha_opt(i));cos(alpha_opt(i));0];
% end
% 
% sign_vec(1,1)=2*a^2/h*dot([ep2*slam-ep1*clam L/r 0],F_sample(:,1));
% sign_vec(2,1)=r/h*dot([-L/r*clam ep1+(1+L/r)*slam -ep2*(zig1*clam-zig2*slam)],F_sample(:,2));
% sign_vec(3,1)=r/h*dot([L/r*slam ep2+(1+L/r)*clam ep1*(zig1*clam-zig2*slam)],F_sample(:,3));
% sign_vec(4,1)=r/(2*h)*dot([0 0 (1+zig1^2+zig2^2)*slam],F_sample(:,4));
% sign_vec(5,1)=r/(2*h)*dot([0 0 (1+zig1^2+zig2^2)*clam],F_sample(:,5));
% sign_vec(6,1)=h/r^2+r/h*dot([0 0 zig2*slam-zig1*clam],F_sample(:,6));
% 
% for i=1:6
%     F_sample(:,i)=[0;cos(beta_opt(i));sin(beta_opt(i))];
% end
% 
% 
% 
% sign_vec(1,2)=2*a^2/h*dot([ep2*slam-ep1*clam L/r 0],F_sample(:,1));
% sign_vec(2,2)=r/h*dot([-L/r*clam ep1+(1+L/r)*slam -ep2*(zig1*clam-zig2*slam)],F_sample(:,2));
% sign_vec(3,2)=r/h*dot([L/r*slam ep2+(1+L/r)*clam ep1*(zig1*clam-zig2*slam)],F_sample(:,3));
% sign_vec(4,2)=r/(2*h)*dot([0 0 (1+zig1^2+zig2^2)*slam],F_sample(:,4));
% sign_vec(5,2)=r/(2*h)*dot([0 0 (1+zig1^2+zig2^2)*clam],F_sample(:,5));
% sign_vec(6,2)=h/r^2+r/h*dot([0 0 zig2*slam-zig1*clam],F_sample(:,6));
% 
% sign_vec=sign(sign_vec);





% sign_mat=zeros(6,3);
% 
% sign_mat(1,:)=[ep2*slam-ep1*clam L/r 0];
% sign_mat(2,:)=[-L/r*clam ep1+(1+L/r)*slam -ep2*(zig1*clam-zig2*slam)];
% sign_mat(3,:)=[L/r*slam ep2+(1+L/r)*clam ep1*(zig1*clam-zig2*slam)];
% sign_mat(4,:)=[0 0 (1+zig1^2+zig2^2)*slam];
% sign_mat(5,:)=[0 0 (1+zig1^2+zig2^2)*clam];
% sign_mat(6,:)=[0 0 zig2*slam-zig1*clam];
% 
% sign_mat=sign(sign_mat);


sign_mat=sign([a_dot_;ep1_dot_;ep2_dot_;zig1_dot_;zig2_dot_;lambda_dot_]);




end

== matlab function model_5_exact/MATLAB Function2 ==
  data: W input; mee_0 input; mee_f input; mee input; alpha_opt input; beta_opt input; T output; R output; stop output; sign_mat input; R_stop input
function [T,R,stop]  = Guider(W,mee_0,mee_f,mee,alpha_opt,beta_opt,sign_mat,R_stop)


stop=0;

% mark=0;

R=zeros(6,1);


%
% ss(1)=-1;
% ss(2)=-1;
% % ss(4)=-1;

T=[0;0;0];

% for i=1:5
%
%     %     if abs(mee_f(i)-mee_0(i))>1e-5 && abs(mee_f(i)-mee(i))>1e-5
%
%     if abs(mee_f(i)-mee_0(i))>1e-5
%
%         R(i)=abs((mee(i)-mee_f(i))/(mee_f(i)-mee_0(i)));
%
%         %         if  abs(R(i))>5
%         %             R(i)=5;
%         %         end
%         %         if  abs(R(i))<-5
%         %             R(i)=-5;
%         %         end
%
%     else
%         R(i)=0;
%     end
% end


for i=1:5

    %     if abs(mee_f(i)-mee_0(i))>1e-5 && abs(mee_f(i)-mee(i))>1e-5
    %      ss(i)=sign(oe_f(i)-oe(i));

    if abs(mee_f(i)-mee_0(i))>1e-5

        R(i)=abs((mee_f(i)-mee(i))/(mee_f(i)-mee_0(i)));

        %         if  abs(R(i))>5
        %             R(i)=5;
        %         end
        %         if  abs(R(i))<-5
        %             R(i)=-5;
        %         end


    else
        R(i)=0;
    end
end



if norm(R)<R_stop
    stop=1;
end

% ss(1)=-1;

% alpha_opt1=zeros(6,1);
% beta_opt1=zeros(6,1);


alpha_opt1=alpha_opt;
beta_opt1=beta_opt;



% % % ss(1)=sign(mee_f(1)-mee(1));  %% sign ok
% % % ss(2)=-sign(mee_f(2)-mee(2));  %% sign ok
% % % ss(3)=-sign(mee_f(3)-mee(3));
% % % ss(4)=sign(mee_f(4)-mee(4));
% % % ss(5)=sign(mee_f(5)-mee(5));
% % % ss(6)=sign(mee_f(6)-mee(6));

% ss=R_dot;

% ang1=rem(x(6)+2*pi,2*pi);
% if ang1>pi
%     ss(2)=-ss(2);
% alpha_opt(2)=2*pi-alpha_opt(2);
% end

% n=0;

%
% if mee_f(1)<mee(1)
%     ss(1)=-1;
% end
%
% if mee_f(2)<mee(2)
%     ss(2)=-1;
% end

% sign_mat1=ones(6,3);

% for i=1:6
%     for j=1:3
%         if (sign_mat(i,j)<0 && mee_f(i)>mee(i)) || (sign_mat(i,j)>0 && mee_f(i)<mee(i))
%             sign_mat1(i,j)=-1;
%         end
%     end
%
% end

% for i=1:6
%         if (sign_vec(i,1)<0 && mee_f(i)>mee(i)) || (sign_vec(i,1)>0 && mee_f(i)<mee(i)) || (sign_vec(i,2)<0 && mee_f(i)>mee(i)) || (sign_vec(i,2)>0 && mee_f(i)<mee(i))
%             ss(i)=-1;
%         end
% 
% end


% for i=1:6
%     if (sign_vec(i,1)<0 && oe_f(i)>oe(i)) || (sign_vec(i,1)>0 && oe_f(i)<oe(i))
%         alpha_opt1(i)= -alpha_opt(i);
%     end
% 
%     if (sign_vec(i,2)<0 && oe_f(i)>oe(i)) || (sign_vec(i,2)>0 && oe_f(i)<oe(i))
%         beta_opt1(i)= -beta_opt(i);
%     end
% end


% for i=1:6
%     if (sign_vec(i,1)<0 && R(i)>0) || (sign_vec(i,1)>0 && R(i)<0)
%         alpha_opt1(i)= -alpha_opt(i);
%     end
% 
%     if (sign_vec(i,2)<0 && R(i)>0) || (sign_vec(i,2)>0 && R(i)<0)
%         beta_opt1(i)= -beta_opt(i);
%     end
% end

% for i=1:5
%     if sign_vec(i,1)<0
%         alpha_opt1(i)= pi+alpha_opt(i);
%     end
% 
%     if sign_vec(i,2)<0
%         beta_opt1(i)= pi+beta_opt(i);
%     end
% end



% for i=1:5
%     s1=0;
%     s2=0;
%     if (sign_vec(i,1)==-1  && mee_f(i)>mee(i)) || (sign_vec(i,1)==1 && mee_f(i)<mee(i))
% %         ss(i)=-1;
%                 alpha_opt1(i)=-alpha_opt1(i);
%         s1=1;
% 
%     end
% 
%     if (sign_vec(i,2)==-1  && mee_f(i)>mee(i)) || (sign_vec(i,2)==1 && mee_f(i)<mee(i))
% %         ss(i)=-1;
%                 beta_opt1(i)=-beta_opt1(i);
%         s2=1;
%     end
% 
%     if s1~=s2
%         mark=1;
%     end
% 
%     %     if (sign_vec(i,2)==-1  && mee_f(i)>mee(i)) || (sign_vec(i,2)==1 && mee_f(i)<mee(i))
%     %         beta_opt1(i)=pi+beta_opt1(i);
%     %     end
% end


ss_rsw=ones(6,3);

for i=1:6
    for j=1:3
        if (sign_mat(i,j)<0 && mee_f(i)>mee(i)) || (sign_mat(i,j)>0 && mee_f(i)<mee(i))
            ss_rsw(i,j)=-1;
        end
    end
end

for i=1:5

    %     n=n+1;
    %     ss=1;
    %     ang1=rem(x(6)+2*pi,2*pi);
    %     if ang1<pi
    %         alpha_opt(i)=-alpha_opt(i);
    % ss=-1;
    %     end

    %         ss=sign(x(i)-mp_f(i));
    %     ss=1;
    %
    % ss=-1;

    %     if (sign_mat(i,1)==-1  && mee_f(i)>mee(i)) || (sign_mat(i,1)==1 && mee_f(i)<mee(i))
    %         alpha_opt(i)=-abs(alpha_opt(i));
    %     else
    %         alpha_opt(i)=abs(alpha_opt(i));
    %     end
    %
    %     if (sign_mat(i,3)==-1  && mee_f(i)>mee(i)) || (sign_mat(i,3)==1 && mee_f(i)<mee(i))
    %         beta_opt(i)=-abs(beta_opt(i));
    %     else
    %         beta_opt(i)=abs(beta_opt(i));
    %     end

    %     if (sign_mat(i,1)==-1  && mee_f(i)>mee(i)) || (sign_mat(i,1)==1 && mee_f(i)<mee(i))
    %                 alpha_opt1(i)=-alpha_opt(i);
    % %         ss(i)=-1;
    %     else
    %                 alpha_opt1(i)=abs(alpha_opt(i));
    %     end
    %
    %     if (sign_mat(i,3)==-1  && mee_f(i)>mee(i)) || (sign_mat(i,3)==1 && mee_f(i)<mee(i))
    %                 beta_opt1(i)=-beta_opt(i);
    %     else
    %                 beta_opt1(i)=abs(beta_opt(i));
    %     end






%     T=T+ss(i)*W(i)*R(i)*([sin(alpha_opt1(i))*cos(beta_opt1(i));cos(alpha_opt1(i))*cos(beta_opt1(i));sin(beta_opt1(i))]);

    T=T+W(i)*R(i)*([ss_rsw(i,1)*abs(sin(alpha_opt1(i))*cos(beta_opt1(i)));ss_rsw(i,2)*abs(cos(alpha_opt1(i))*cos(beta_opt1(i)));ss_rsw(i,3)*abs(sin(beta_opt1(i)))]);

    % T=T+ss(n)*W(n)*R(i)*([sin(alpha_opt(i))*cos(0);cos(alpha_opt(i))*cos(0);sin(beta_opt(i))]);
    %
end

% for i=1:6
%     n=n+1;
%     ss=1;
%     ang1=rem(x(6)+2*pi,2*pi);
%     if ang1<pi
%         alpha_opt(i)=-alpha_opt(i);
% ss=-1;
%     end

%         ss=sign(x(i)-mp_f(i));
%     ss=1;
%
% ss=-1;
%     T=T+ss(i)*W(i)*R(i)*([sin(alpha_opt(i))*cos(beta_opt(i));cos(alpha_opt(i))*cos(beta_opt(i));sin(beta_opt(i))]);
% T=T+ss(i)*W(n)*R(i)*([sin(0)*cos(beta_opt(i));cos(0)*cos(beta_opt(i));sin(beta_opt(i))]);
%
% end

% T=T./sum(W);


T=T./sum(W);


% if norm(T)>1e-10
% 
%     T=T./norm(T);
% 
% else
%     T=[0;0;0];
% end

end

== matlab function model_5_exact/Subsystem1/MATLAB Function3 ==
  data: mp input; oe output; mu input; r output; v output
function [oe,r,v]=mp2oe(mp,mu)



oe=mp2oe(mp);

[r, v] = oe2rv(oe,mu);



% % % % a=mp(1);
% % % % ep1=mp(2);
% % % % ep2=mp(3);
% % % % zig1=mp(4);
% % % % zig2=mp(5);
% % % % lambda=mp(6);
% % % % 
% % % % 
% % % % % % ep1=e*sin(omega+OMEGA);
% % % % % % ep2=e*cos(omega+OMEGA);
% % % % % % zig1=tan(inc/2)*sin(OMEGA);
% % % % % % zig2=tan(inc/2)*cos(OMEGA);
% % % % % % lambda=theta+omega+OMEGA;
% % % % % %
% % % % % % mp=[a;ep1;ep2;zig1;zig2;lambda];
% % % % 
% % % % %%% to be optimized
% % % % e=sqrt(ep1^2+ep2^2);
% % % % inc=2*atan(sqrt(zig1^2+zig2^2));
% % % % 
% % % % if inc==0
% % % %     OMEGA=0;
% % % % else
% % % %     tan1=tan(inc/2);
% % % %     OMEGA=atan3(zig1/tan1,zig2/tan1);
% % % % end
% % % % 
% % % % 
% % % % % if sign(zig2)*sign(cos(OMEGA))<0 || sign(zig1)*sign(sin(OMEGA))<0
% % % % %     inc=-inc;
% % % % % end
% % % % 
% % % % 
% % % % if OMEGA>pi
% % % %     OMEGA=OMEGA-2*pi;
% % % % end
% % % % 
% % % % % inc=inc*(sign(zig2)*sign(cos(OMEGA)));
% % % % 
% % % % if e==0
% % % %     omega=0;
% % % % else
% % % %     omega=atan3(ep1/e,ep2/e)-OMEGA;
% % % % end
% % % % 
% % % % if omega>2*pi
% % % %     omega=omega-2*pi;
% % % %     
% % % % end
% % % % 
% % % % 
% % % % theta=lambda-omega-OMEGA;
% % % % if theta<0
% % % %     theta=theta+2*pi;
% % % % end
% % % % 
% % % % if theta>2*pi
% % % %     theta=rem(theta,2*pi);
% % % % end
% % % % 
% % % % oe=[a;e;inc;omega;OMEGA;theta];


end

== matlab function model_5_exact/Subsystem/Subsystem1/MATLAB Function ==
  data: A input; delta output
function delta = fcn(A)

delta=zeros(3,1);

delta(1)=0.5*(A(2,3)-A(3,2));
delta(2)=0.5*(A(3,1)-A(1,3));
delta(3)=0.5*(A(1,2)-A(2,1));


end

== matlab function model_5_exact/Subsystem/rsw 2 B/MATLAB Function5 ==
  data: Vector_rsw input; R input; Vector_xyz output; V input
function Vector_xyz=rsw2xyz(Vector_rsw,R,V)



e_r=R/norm(R);
h=cross(R,V);
e_w=h/norm(h);
e_s=cross(e_w,e_r);


Vector_xyz=Vector_rsw(1)*e_r+Vector_rsw(2)*e_s+Vector_rsw(3)*e_w;


end
